simulink model "threephaseinverter_mosfet_model"  (R2026a)
settings: Solver=VariableStepAuto  StopTime=0.3
undefined symbols (not defined in the file): fout, fsw, ModIndex, Rload, Vg
libraries: fl_lib x41, nesl_utility x37, ee_lib x10, simulink x1
(part 2 of 2)

== matlab function threephaseinverter_mosfet_model/MATLAB Function1 ==
  data: G3raw input; G3 output; G4raw input; Ndead input; G4 output
function [G3, G4] = deadtime_G3G4(G3raw, G4raw, Ndead)

persistent G3_state G4_state cnt3 cnt4

if isempty(G3_state)
    G3_state = false;
    G4_state = false;
    cnt3 = 0;
    cnt4 = 0;
end

G3raw = logical(G3raw);
G4raw = logical(G4raw);
Ndead = max(0, round(Ndead));

if G3raw && G4raw
    G3_state = false;
    G4_state = false;
    cnt3 = 0;
    cnt4 = 0;

elseif G3raw
    G4_state = false;
    cnt4 = 0;

    if cnt3 >= Ndead
        G3_state = true;
    else
        G3_state = false;
        cnt3 = cnt3 + 1;
    end

elseif G4raw
    G3_state = false;
    cnt3 = 0;

    if cnt4 >= Ndead
        G4_state = true;
    else
        G4_state = false;
        cnt4 = cnt4 + 1;
    end

else
    G3_state = false;
    G4_state = false;
    cnt3 = 0;
    cnt4 = 0;
end

G3 = G3_state;
G4 = G4_state;

end

== matlab function threephaseinverter_mosfet_model/MATLAB Function ==
  data: G1raw input; G1 output; G2raw input; Ndead input; G2 output
function [G1, G2] = deadtime_G1G2(G1raw, G2raw, Ndead)

persistent G1_state G2_state cnt1 cnt2

if isempty(G1_state)
    G1_state = false;
    G2_state = false;
    cnt1 = 0;
    cnt2 = 0;
end

G1raw = logical(G1raw);
G2raw = logical(G2raw);
Ndead = max(0, round(Ndead));

if G1raw && G2raw
    G1_state = false;
    G2_state = false;
    cnt1 = 0;
    cnt2 = 0;

elseif G1raw
    G2_state = false;
    cnt2 = 0;

    if cnt1 >= Ndead
        G1_state = true;
    else
        G1_state = false;
        cnt1 = cnt1 + 1;
    end

elseif G2raw
    G1_state = false;
    cnt1 = 0;

    if cnt2 >= Ndead
        G2_state = true;
    else
        G2_state = false;
        cnt2 = cnt2 + 1;
    end

else
    G1_state = false;
    G2_state = false;
    cnt1 = 0;
    cnt2 = 0;
end

G1 = G1_state;
G2 = G2_state;

end

== matlab function threephaseinverter_mosfet_model/MATLAB Function2 ==
  data: G5raw input; G5 output; G6raw input; Ndead input; G6 output
function [G5, G6] = deadtime_G5G6(G5raw, G6raw, Ndead)

persistent G5_state G6_state cnt5 cnt6

if isempty(G5_state)
    G5_state = false;
    G6_state = false;
    cnt5 = 0;
    cnt6 = 0;
end

G5raw = logical(G5raw);
G6raw = logical(G6raw);
Ndead = max(0, round(Ndead));

if G5raw && G6raw
    G5_state = false;
    G6_state = false;
    cnt5 = 0;
    cnt6 = 0;

elseif G5raw
    G6_state = false;
    cnt6 = 0;

    if cnt5 >= Ndead
        G5_state = true;
    else
        G5_state = false;
        cnt5 = cnt5 + 1;
    end

elseif G6raw
    G5_state = false;
    cnt5 = 0;

    if cnt6 >= Ndead
        G6_state = true;
    else
        G6_state = false;
        cnt6 = cnt6 + 1;
    end

else
    G5_state = false;
    G6_state = false;
    cnt5 = 0;
    cnt6 = 0;
end

G5 = G5_state;
G6 = G6_state;

end
